simulink model "LCK_0112"  (R2018b)
settings: Solver=FixedStepDiscrete  StartTime=0.0  StopTime=inf  FixedStep=0.01  RelTol=1e-3
PostLoadFcn:
  | if any(exist('dsrtsu_mdlpostloadfcn', 'file') ~= 0), dsrtsu_mdlpostloadfcn('Execute', bdroot); end
values from neighbouring files (symbols this model uses):
  C_DEG2RAD = 0.0175    [LCK_Macro.sldd]
  C_KPH2MPS = 0.2778    [LCK_Macro.sldd]
  C_NEARZERO = 0.0001    [LCK_Macro.sldd]
  C_ONE = 1.0    [LCK_Macro.sldd]
  C_RAD2DEG = 57.2958    [LCK_Macro.sldd]
  C_ZERO = 0.0    [LCK_Macro.sldd]
  k_accel_pedal_pos_per_speed_x : value not decoded    [LCK_LogicPara.sldd]
  k_accel_pedal_pos_per_speed_z : value not decoded    [LCK_LogicPara.sldd]
  k_brake_suprress_hold = 1000.0    [LCK_LogicPara.sldd]
  k_driver_appl_torque_filt = 50.0    [LCK_LogicPara.sldd]
  k_driver_suppression_hold_time = 3000.0    [LCK_LogicPara.sldd]
  k_hands_on_wheel_hold_msec = 500.0    [LCK_LogicPara.sldd]
  k_hands_on_wheel_torque_hi = 0.2    [LCK_LogicPara.sldd]
  k_hands_on_wheel_torque_lo = 0.15    [LCK_LogicPara.sldd]
  k_handsoff_delay_cycles = 50.0    [LCK_LogicPara.sldd]
  k_handsoff_torq_Lo_CR = 0.3    [LCK_LogicPara.sldd]
  k_handson_delay_cycles = 5.0    [LCK_LogicPara.sldd]
  k_HighAccel_suppress_hold = 3000.0    [LCK_LogicPara.sldd]
  k_HLR_suprress_hold = 3000.0    [LCK_LogicPara.sldd]
  k_hs_StrAng_CR_threshold_z : value not decoded    [LCK_LogicPara.sldd]
  k_LC_Exit_Switch = 0.0    [LCK_LogicPara.sldd]
  k_LCG_Configured = 1.0    [LCK_LogicPara.sldd]
  k_LCK_A0_Rdy2Act_UseConst = 0.0    [LCK_LogicPara.sldd]
  k_LCK_A0Fac_ActSta : value not decoded    [LCK_CtrlPara.sldd]
  k_LCK_A0Fac_DrvStm : value not decoded    [LCK_CtrlPara.sldd]
  k_LCK_A0Shift_LftCurv : value not decoded    [LCK_CtrlPara.sldd]
  k_LCK_A0Shift_RgtCurv : value not decoded    [LCK_CtrlPara.sldd]
  k_LCK_A0Shift_StraLan = 0.0    [LCK_CtrlPara.sldd]
  k_LCK_A0ShiftFac_Dy_LftCurv : value not decoded    [LCK_CtrlPara.sldd]
  k_LCK_A0ShiftFac_Dy_RgtCurv : value not decoded    [LCK_CtrlPara.sldd]
  k_LCK_A0ShiftFac_Vspd : value not decoded    [LCK_CtrlPara.sldd]
  k_LCK_accel_inhibit_thold = 35.0    [LCK_LogicPara.sldd]
  k_LCK_Active2Ready_Mask = 255.0    [LCK_LogicPara.sldd]
  k_LCK_CvatRateBks : value not decoded    [LCK_CtrlPara.sldd]
  k_LCK_CvatrBks : value not decoded    [LCK_CtrlPara.sldd]
  k_LCK_DFac_Dy : value not decoded    [LCK_CtrlPara.sldd]
  k_LCK_DFac_Dy_Curv : value not decoded    [LCK_CtrlPara.sldd]
  k_LCK_DFac_HaCurCen : value not decoded    [LCK_CtrlPara.sldd]
  k_LCK_DFac_HaCurSid : value not decoded    [LCK_CtrlPara.sldd]
  k_LCK_DFac_HadCurCen : value not decoded    [LCK_CtrlPara.sldd]
  k_LCK_DFac_HadCurSid : value not decoded    [LCK_CtrlPara.sldd]
  k_LCK_DFac_HadStrCen : value not decoded    [LCK_CtrlPara.sldd]
  k_LCK_DFac_HadStrSid : value not decoded    [LCK_CtrlPara.sldd]
  k_LCK_DFac_HaStrCen : value not decoded    [LCK_CtrlPara.sldd]
  k_LCK_DFac_HaStrSid : value not decoded    [LCK_CtrlPara.sldd]
  k_LCK_DFac_Rad : value not decoded    [LCK_CtrlPara.sldd]
  k_LCK_DFac_SA_CurCen : value not decoded    [LCK_CtrlPara.sldd]
  k_LCK_DFac_SA_CurSid : value not decoded    [LCK_CtrlPara.sldd]
  k_LCK_DFac_SA_StrCen : value not decoded    [LCK_CtrlPara.sldd]
  k_LCK_DFac_SA_StrSid : value not decoded    [LCK_CtrlPara.sldd]
  k_LCK_DFac_SS_CurCen : value not decoded    [LCK_CtrlPara.sldd]
  k_LCK_DFac_SS_CurSid : value not decoded    [LCK_CtrlPara.sldd]
  k_LCK_DFac_SS_StrCen : value not decoded    [LCK_CtrlPara.sldd]
  k_LCK_DFac_SS_StrSid : value not decoded    [LCK_CtrlPara.sldd]
  k_LCK_DFac_Vspd : value not decoded    [LCK_CtrlPara.sldd]
  k_LCK_DlyTm_DrvStim = 0.2    [LCK_CtrlPara.sldd]
  k_LCK_DTermMax = 2.0    [LCK_CtrlPara.sldd]
  k_LCK_DyBks_Curv : value not decoded    [LCK_CtrlPara.sldd]
  k_LCK_Enable_POOnly = 1.0    [LCK_LogicPara.sldd]
  k_LCK_Entry_DistBuffer = 0.1    [LCK_LogicPara.sldd]
  k_LCK_Fac_Vspd2RngThr_FalRec = 0.23    [LCK_CtrlPara.sldd]
  k_LCK_Ffw_CvatSwh = 0.0    [LCK_CtrlPara.sldd]
  k_LCK_Ffw_DyBks : value not decoded    [LCK_CtrlPara.sldd]
  k_LCK_Ffw_TimCon_CmdFlt = 0.0    [LCK_CtrlPara.sldd]
  k_LCK_FfwDeltaFac_Rad_Lft : value not decoded    [LCK_CtrlPara.sldd]
  k_LCK_FfwDeltaFac_Rad_Rgt : value not decoded    [LCK_CtrlPara.sldd]
  k_LCK_FfwDeltaFac_Vspd : value not decoded    [LCK_CtrlPara.sldd]
  k_LCK_FfwFac_CvatRate_Lft : value not decoded    [LCK_CtrlPara.sldd]
  k_LCK_FfwFac_CvatRate_Rgt : value not decoded    [LCK_CtrlPara.sldd]
  k_LCK_FfwFac_Dy : value not decoded    [LCK_CtrlPara.sldd]
  k_LCK_FfwFac_Rad_Lft : value not decoded    [LCK_CtrlPara.sldd]
  k_LCK_FfwFac_Rad_Rgt : value not decoded    [LCK_CtrlPara.sldd]
  k_LCK_FfwFac_Vspd : value not decoded    [LCK_CtrlPara.sldd]
  k_LCK_FfwTorq_Cvat : value not decoded    [LCK_CtrlPara.sldd]
  k_LCK_HAFac_ActSta : value not decoded    [LCK_CtrlPara.sldd]
  k_LCK_HAFac_DrvStm : value not decoded    [LCK_CtrlPara.sldd]
  k_LCK_HaloTime = 2000.0    [LCK_LogicPara.sldd]
  k_LCK_HaloTime_Switch = 0.0    [LCK_LogicPara.sldd]
  k_LCK_HARFac_ActSta : value not decoded    [LCK_CtrlPara.sldd]
  k_LCK_HARFac_DrvStm : value not decoded    [LCK_CtrlPara.sldd]
  k_LCK_Hed_DyBks : value not decoded    [LCK_CtrlPara.sldd]
  k_LCK_HedAngDiffX : value not decoded    [LCK_CtrlPara.sldd]
  k_LCK_HedAngRateDiffX : value not decoded    [LCK_CtrlPara.sldd]
  k_LCK_HndsOnWhel_DlyTm_Idl2Rdy = 0.0    [LCK_LogicPara.sldd]
  k_LCK_host_veh_width = 1.86    [LCK_LogicPara.sldd]
  k_LCK_Idle2Ready_Mask = 239.0    [LCK_LogicPara.sldd]
  k_LCK_Junc_SusTime = 1.0    [LCK_LogicPara.sldd]
  k_LCK_KpKdDecSlopeLmt = 10.0    [LCK_CtrlPara.sldd]
  k_LCK_KpKdIncSlopeLmt = 5.0    [LCK_CtrlPara.sldd]
  k_LCK_Lat_Ctrl_DFac_Lft = 1.0    [LCK_CtrlPara.sldd]
  k_LCK_Lat_Ctrl_DFac_Rgt = 1.05    [LCK_CtrlPara.sldd]
  k_LCK_Lat_Ctrl_Kd = 0.8    [LCK_CtrlPara.sldd]
  k_LCK_Lat_Ctrl_Ki = 0.5    [LCK_CtrlPara.sldd]
  k_LCK_Lat_Ctrl_Kp = 0.7    [LCK_CtrlPara.sldd]
  k_LCK_Lat_Ctrl_Kp_NearGain = 0.7    [LCK_CtrlPara.sldd]
  k_LCK_Lat_Ctrl_PFac_Lft = 1.0    [LCK_CtrlPara.sldd]
  k_LCK_Lat_Ctrl_PFac_Rgt = 1.05    [LCK_CtrlPara.sldd]
  k_LCK_Lat_Ctrl_TimCon_CmdFlt = 5.0    [LCK_CtrlPara.sldd]
  k_LCK_Lat_DFac_Rad : value not decoded    [LCK_CtrlPara.sldd]
  k_LCK_Lat_DFac_SS_Cur : value not decoded    [LCK_CtrlPara.sldd]
  k_LCK_Lat_DFac_SS_Str : value not decoded    [LCK_CtrlPara.sldd]
  k_LCK_Lat_DFac_Vspd : value not decoded    [LCK_CtrlPara.sldd]
  k_LCK_Lat_DyBks : value not decoded    [LCK_CtrlPara.sldd]
  k_LCK_Lat_IFac_Rad : value not decoded    [LCK_CtrlPara.sldd]
  k_LCK_Lat_IFac_Vspd : value not decoded    [LCK_CtrlPara.sldd]
  k_LCK_Lat_ILmtFac_Dy_CurvLan : value not decoded    [LCK_CtrlPara.sldd]
  k_LCK_Lat_ILmtFac_Dy_StraLan : value not decoded    [LCK_CtrlPara.sldd]
  k_LCK_Lat_ILmtFac_Rad : value not decoded    [LCK_CtrlPara.sldd]
  k_LCK_Lat_ILmtFac_Rad_NearGain = 1.0    [LCK_CtrlPara.sldd]
  k_LCK_Lat_ILmtFac_Vspd_CurvLan : value not decoded    [LCK_CtrlPara.sldd]
  k_LCK_Lat_ILmtFac_Vspd_StraLan : value not decoded    [LCK_CtrlPara.sldd]
  k_LCK_Lat_ITermLmt_Dy = 1.0    [LCK_CtrlPara.sldd]
  k_LCK_Lat_KpKdDecSlopeLmt = 10.0    [LCK_CtrlPara.sldd]
  k_LCK_Lat_KpKdIncSlopeLmt = 10.0    [LCK_CtrlPara.sldd]
  k_LCK_Lat_PFac_Dy_InnLftCur : value not decoded    [LCK_CtrlPara.sldd]
  k_LCK_Lat_PFac_Dy_InnRgtCur : value not decoded    [LCK_CtrlPara.sldd]
  k_LCK_Lat_PFac_Dy_OutLftCur : value not decoded    [LCK_CtrlPara.sldd]
  k_LCK_Lat_PFac_Dy_OutRgtCur : value not decoded    [LCK_CtrlPara.sldd]
  k_LCK_Lat_PFac_Dy_Str : value not decoded    [LCK_CtrlPara.sldd]
  k_LCK_Lat_PFac_Rad : value not decoded    [LCK_CtrlPara.sldd]
  ... (+153 more)
undefined symbols (not defined in the file or in its folder): k_LCK_CurvBks, K_LCK_SPA0A1A2_LMRngCmp_y
libraries: LateralControl_fcns_lib x58, simulink x24
(part 38 of 45)

== system LCK_0112/Lateral_Control_Module/Adas_Lateral_Control_LCK_Core/Module 8/Module 0/Limitation of P1 Gain ==
  P1_Gain : Inport  Description=_GWMH9P2.LKAFN.000_2_
  Gain : Gain  Description=_GWMH9P2.LKAFN.000_5_  Gain=ML_TIME_MSEC
  Gain1 : Gain  Description=_GWMH9P2.LKAFN.000_6_  Gain=ML_TIME_MSEC
  Gain2 : Gain  Description=_GWMH9P2.LKAFN.000_7_  Gain=-1
  Product3 : Product  Description=_GWMH9P2.LKAFN.000_8_  Inputs=*/  OutDataTypeStr=Inherit: Same as first input
  Product5 : Product  Description=_GWMH9P2.LKAFN.000_9_  Inputs=*/  OutDataTypeStr=Inherit: Same as first input
  Relational Operator1 : RelationalOperator  Description=_GWMH9P2.LKAFN.000_11_  Operator=<  RndMeth=Nearest
  Relational Operator4 : RelationalOperator  Description=_GWMH9P2.LKAFN.000_12_  Operator=>  RndMeth=Nearest
  Sum : Sum  Description=_GWMH9P2.LKAFN.000_13_  Inputs=+-  InputSameDT=on  OutDataTypeStr=Inherit: Same as first input
  Sum1 : Sum  Description=_GWMH9P2.LKAFN.000_14_  InputSameDT=on  OutDataTypeStr=Inherit: Same as first input
  Switch19 : Switch  Description=_GWMH9P2.LKAFN.000_15_  Threshold=0.5  OutDataTypeStr=Inherit: Inherit via back propagation
  Switch20 : Switch  Description=_GWMH9P2.LKAFN.000_16_  Threshold=0.5  OutDataTypeStr=Inherit: Inherit via back propagation
  Unit Delay : UnitDelay  Description=_GWMH9P2.LKAFN.000_17_  SampleTime=-1
  const : Constant  Description=_GWMH9P2.LKAFN.000_18_  Value=1000  OutDataTypeStr=uint16
  const1 : Constant  Description=_GWMH9P2.LKAFN.000_19_  Value=1000  OutDataTypeStr=uint16
  k_LCK_Lat_KpKdDecSlopeLmt : Constant  Description=_GWMAB30P3.LCK.000_168_  Value=k_LCK_Lat_KpKdDecSlopeLmt
  k_LCK_Lat_KpKdIncSlopeLmt : Constant  Description=_GWMAB30P3.LCK.000_168_  Value=k_LCK_Lat_KpKdIncSlopeLmt
  P1_Gain_Limited : Outport  Description=_GWMH9P2.LKAFN.000_32_
  wires:
  Switch19/1 -> Relational Operator4/2, Switch20/3
  Product3/1 -> Relational Operator4/1, Switch20/1
  const1/1 -> Product5/2
  Relational Operator1/1 -> Switch19/2
  Gain2/1 -> Gain/1
  k_LCK_Lat_KpKdIncSlopeLmt/1 -> Gain1/1
  const/1 -> Product3/2
  Gain1/1 -> Product5/1
  P1_Gain/1 -> Sum/1
  Unit Delay/1 -> Sum/2, Sum1/2
  k_LCK_Lat_KpKdDecSlopeLmt/1 -> Gain2/1
  Switch20/1 -> Sum1/1
  Sum1/1 -> P1_Gain_Limited/1, Unit Delay/1
  Relational Operator4/1 -> Switch20/2
  Gain/1 -> Product3/1
  Product5/1 -> Relational Operator1/1, Switch19/1
  Sum/1 -> Relational Operator1/2, Switch19/3

== system LCK_0112/Lateral_Control_Module/Adas_Lateral_Control_LCK_Core/Module 8/Module 0/P0 Gain ==
  LatCtrl_P0Fac_Asym : Inport
  LatCtrl_P0Fac_Dy : Inport  Port=2
  LatCtrl_PFac_Vspd : Inport  Port=3
  LatCtrl_PFac_Radius : Inport  Port=4
  LatCtrl_PFac_StrSpd : Inport  Port=5
  Gain : Gain  Gain=2
  Product : Product  Inputs=6
  Product6 : Product
  k_LCK_Lat_Ctrl_Kp : Constant  Value=k_LCK_Lat_Ctrl_Kp
  k_LCK_Lat_Ctrl_Kp_NearGain : Constant  Value=k_LCK_Lat_Ctrl_Kp_NearGain
  P0_Gain : Outport
  wires:
  Product/1 -> P0_Gain/1
  LatCtrl_P0Fac_Asym/1 -> Product/2
  LatCtrl_P0Fac_Dy/1 -> Product/3
  LatCtrl_PFac_Vspd/1 -> Product/4
  LatCtrl_PFac_Radius/1 -> Product/5
  LatCtrl_PFac_StrSpd/1 -> Product/6
  k_LCK_Lat_Ctrl_Kp_NearGain/1 -> Product6/2
  k_LCK_Lat_Ctrl_Kp/1 -> Product6/1
  Product6/1 -> Gain/1
  Gain/1 -> Product/1

== system LCK_0112/Lateral_Control_Module/Adas_Lateral_Control_LCK_Core/Module 8/Module 0/P1 Gain ==
  LatCtrl_P1Fac_Asym : Inport
  LatCtrl_P1Fac_Dy : Inport  Port=2
  LatCtrl_PFac_Vspd : Inport  Port=3
  LatCtrl_PFac_Radius : Inport  Port=4
  LatCtrl_PFac_StrSpd : Inport  Port=5
  Gain : Gain  Gain=2
  Product : Product  Inputs=6
  k_LCK_Lat_Ctrl_Kp : Constant  Value=k_LCK_Lat_Ctrl_Kp
  P1_Gain : Outport
  wires:
  k_LCK_Lat_Ctrl_Kp/1 -> Gain/1
  LatCtrl_PFac_StrSpd/1 -> Product/6
  LatCtrl_PFac_Radius/1 -> Product/5
  LatCtrl_PFac_Vspd/1 -> Product/4
  LatCtrl_P1Fac_Dy/1 -> Product/3
  LatCtrl_P1Fac_Asym/1 -> Product/2
  Product/1 -> P1_Gain/1
  Gain/1 -> Product/1

== system LCK_0112/Lateral_Control_Module/Adas_Lateral_Control_LCK_Core/Module 9/Module 0/D Gain ==
  LatCtrl_DFac_Asym : Inport
  LatCtrl_DFac_HedAngDiff : Inport  Port=2
  LatCtrl_DFac_HedAngDiffRat : Inport  Port=3
  LatCtrl_DFac_StrAng : Inport  Port=4
  LatCtrl_DFac_StrSpd : Inport  Port=5
  LatCtrl_DFac_Dy : Inport  Port=6
  LatCtrl_DFac_Vspd : Inport  Port=7
  LatCtrl_DFac_Radius : Inport  Port=8
  Product : Product  Inputs=9
  k_LCK_LatCtrl_Kd : Constant  Value=k_LCK_LatCtrl_Kd
  D_Gain : Outport
  wires:
  LatCtrl_DFac_Radius/1 -> Product/9
  LatCtrl_DFac_StrSpd/1 -> Product/6
  LatCtrl_DFac_Vspd/1 -> Product/8
  LatCtrl_DFac_Asym/1 -> Product/2
  LatCtrl_DFac_HedAngDiff/1 -> Product/3
  k_LCK_LatCtrl_Kd/1 -> Product/1
  Product/1 -> D_Gain/1
  LatCtrl_DFac_HedAngDiffRat/1 -> Product/4
  LatCtrl_DFac_StrAng/1 -> Product/5
  LatCtrl_DFac_Dy/1 -> Product/7

== system LCK_0112/Lateral_Control_Module/Adas_Lateral_Control_LCK_Core/Module 9/Module 0/Definition Fac 1  ==
  Hed_Ang : Inport
  Hed_Ang_Diff_Rat : Inport  Port=2
  Relay : Relay  OnSwitchValue=0.05  OffSwitchValue=-0.05
  Relay1 : Relay  OnSwitchValue=0.05  OffSwitchValue=-0.05
  Switch25 : Switch  Criteria=u2 > Threshold
  Switch26 : Switch  Criteria=u2 > Threshold
  k_LCK_LatCtrl_DFac_Lft : Constant  Value=k_LCK_LatCtrl_DFac_Lft
  k_LCK_LatCtrl_DFac_Rgt : Constant  Value=k_LCK_LatCtrl_DFac_Rgt
  k_LCK_LatCtrl_PFac_Lft : Constant  Value=k_LCK_LatCtrl_PFac_Lft
  k_LCK_LatCtrl_PFac_Rgt : Constant  Value=k_LCK_LatCtrl_PFac_Rgt
  LatCtrl_PFac_Asym : Outport
  LatCtrl_DFac_Asym : Outport  Port=2
  wires:
  Switch26/1 -> LatCtrl_DFac_Asym/1
  k_LCK_LatCtrl_DFac_Rgt/1 -> Switch26/1
  Relay/1 -> Switch25/2
  k_LCK_LatCtrl_DFac_Lft/1 -> Switch26/3
  Hed_Ang/1 -> Relay/1
  k_LCK_LatCtrl_PFac_Rgt/1 -> Switch25/1
  k_LCK_LatCtrl_PFac_Lft/1 -> Switch25/3
  Relay1/1 -> Switch26/2
  Switch25/1 -> LatCtrl_PFac_Asym/1
  Hed_Ang_Diff_Rat/1 -> Relay1/1
